simulink model "HW_P3_8slx"  (R2014a)
settings: Solver=ode45  StartTime=0.0  StopTime=0.05  RelTol=1e-3
settings Model: Creator=pengpeng  LastModifiedBy=pengpeng

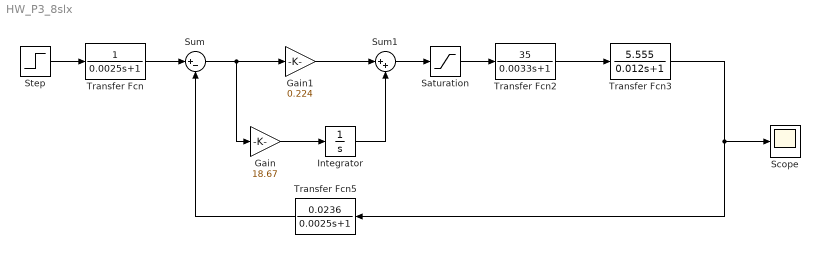
== system HW_P3_8slx ==
  Gain : Gain  Gain=18.67
  Gain1 : Gain  Gain=0.224
  Integrator : Integrator  LimitOutput=on  UpperSaturationLimit=10  LowerSaturationLimit=-10
  Saturation : Saturate  UpperLimit=10  LowerLimit=-10
  Scope : Scope
      settings: TimeRange=2
  Step : Step  Before=1  After=10  SampleTime=0
  Sum : Sum  Inputs=|+-
  Sum1 : Sum  Inputs=|++
  Transfer Fcn : TransferFcn  Denominator=[0.0025 1]
  Transfer Fcn2 : TransferFcn  Numerator=[35]  Denominator=[0.0033 1]
  Transfer Fcn3 : TransferFcn  Numerator=[5.555]  Denominator=[0.012 1]
  Transfer Fcn5 : TransferFcn  Numerator=[0.0236]  Denominator=[0.0025 1]
  wires:
  Step/1 -> Transfer Fcn/1
  Transfer Fcn/1 -> Sum/1
  Sum/1 -> Gain1/1, Gain/1
  Gain/1 -> Integrator/1
  Gain1/1 -> Sum1/1
  Integrator/1 -> Sum1/2
  Transfer Fcn2/1 -> Transfer Fcn3/1
  Sum1/1 -> Saturation/1
  Saturation/1 -> Transfer Fcn2/1
  Transfer Fcn3/1 -> Transfer Fcn5/1, Scope/1
  Transfer Fcn5/1 -> Sum/2
